simulink model "ABS_System"  (R2026a)
settings: Solver=ode4  FixedStep=0.001
undefined symbols (not defined in the file): ABS_MODE, Ts, v0
settings Model: Creator=anh  LastModifiedBy=anh

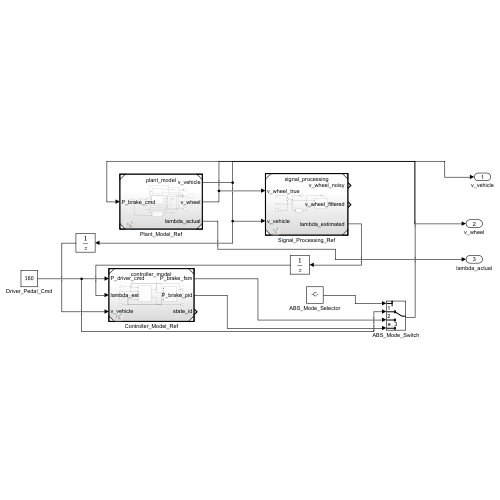
[thumbnail: Simulink's stored preview of the top-level diagram]
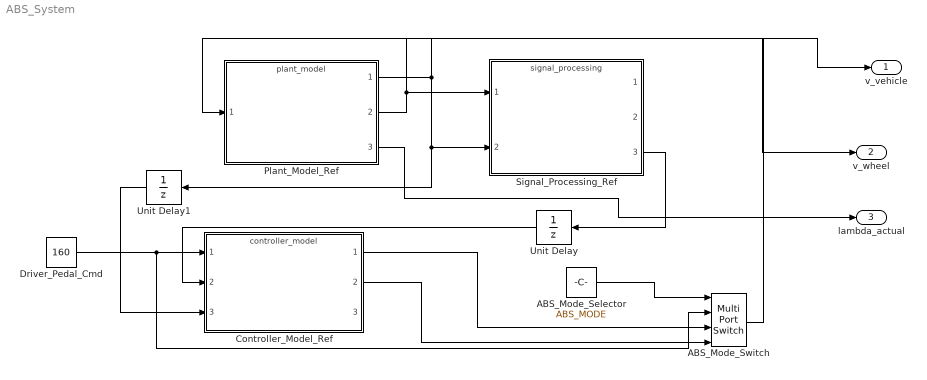
== system ABS_System ==
  ABS_Mode_Selector : Constant  Value=ABS_MODE
  ABS_Mode_Switch : MultiPortSwitch  SaturateOnIntegerOverflow=off  InputSameDT=off
  Controller_Model_Ref : ModelReference  ModelNameDialog=controller_model.slx  SimulationMode=Normal  ModelReferenceVersion=1.6
  Driver_Pedal_Cmd : Constant  Value=160
  Plant_Model_Ref : ModelReference  ModelNameDialog=plant_model.slx  SimulationMode=Normal  ModelReferenceVersion=1.8
  Signal_Processing_Ref : ModelReference  ModelNameDialog=signal_processing.slx  SimulationMode=Normal  ModelReferenceVersion=1.4
  Unit Delay : UnitDelay  SampleTime=Ts
  Unit Delay1 : UnitDelay  InitialCondition=v0  SampleTime=Ts
  v_vehicle : Outport
  v_wheel : Outport  Port=2
  lambda_actual : Outport  Port=3
  wires:
  ABS_Mode_Selector/1 -> ABS_Mode_Switch/1
  Driver_Pedal_Cmd/1 -> Controller_Model_Ref/1, ABS_Mode_Switch/2
  Controller_Model_Ref/1 -> ABS_Mode_Switch/3
  Controller_Model_Ref/2 -> ABS_Mode_Switch/4
  ABS_Mode_Switch/1 -> Plant_Model_Ref/1
  Plant_Model_Ref/2 -> v_wheel/1, Signal_Processing_Ref/1
  Plant_Model_Ref/1 -> v_vehicle/1, Unit Delay1/1, Signal_Processing_Ref/2
  Signal_Processing_Ref/3 -> Unit Delay/1
  Unit Delay/1 -> Controller_Model_Ref/2
  Unit Delay1/1 -> Controller_Model_Ref/3
  Plant_Model_Ref/3 -> lambda_actual/1
